simulink model "bloques_motor"  (R2021b)
settings: Solver=FixedStepAuto  StartTime=0.0  StopTime=Tc  FixedStep=Ts  RelTol=1e-3
values from neighbouring files (symbols this model uses):
  a = (Ts/tau) * Kc    (= 0.000110235109441)    [raiz.m]
  a1 = kp + (ki*Tz)    (= 0.0012908137)    [raiz.m]
  b = (Ts/tau) - 1.0    (= -0.999889764891)    [raiz.m]
  b1 = -kp    (= -0.0012852)    [raiz.m]
  Kc = 1.0    (= 1)    [raiz.m]
  sp = -3000    [raiz.m]
  tau = 0.453576    [raiz.m]
  Tz = 0.001    [raiz.m]
settings Model: Creator=yeezvs  LastModifiedBy=yeezvs
settings DataIOCC: ReturnWorkspaceOutputs=off

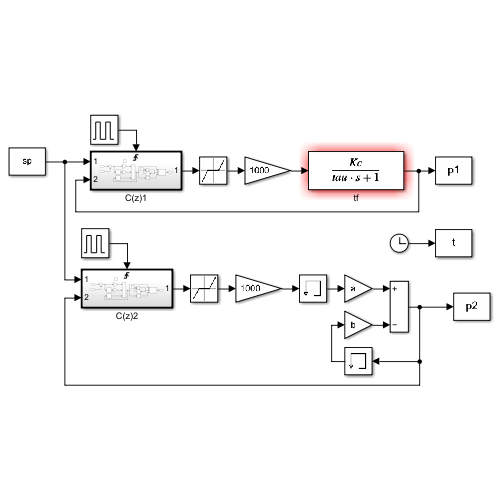
[thumbnail: Simulink's stored preview of the top-level diagram]
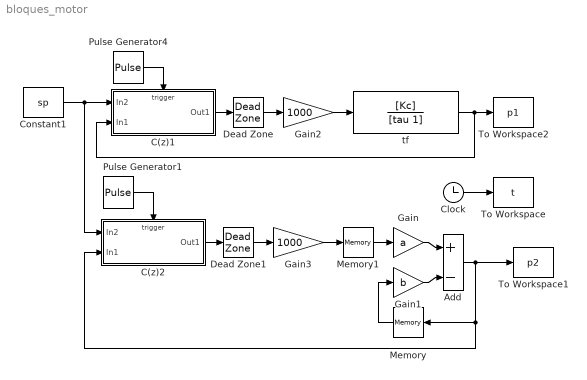
== system bloques_motor ==
  Add : Sum  Inputs=+|-
  C(z)1 : Subsystem  TreatAsAtomicUnit=on
  C(z)2 : Subsystem  TreatAsAtomicUnit=on
  Clock : Clock
  Constant1 : Constant  Value=sp
  Dead Zone : DeadZone  SaturateOnIntegerOverflow=on
  Dead Zone1 : DeadZone  SaturateOnIntegerOverflow=on
  Gain : Gain  Gain=a
  Gain1 : Gain  Gain=b
  Gain2 : Gain  Gain=1000
  Gain3 : Gain  Gain=1000
  Memory : Memory
  Memory1 : Memory
  Pulse Generator1 : DiscretePulseGenerator  PulseType=Time based  Period=Tz  PulseWidth=50
  Pulse Generator4 : DiscretePulseGenerator  PulseType=Time based  Period=Tz  PulseWidth=50
  To Workspace : ToWorkspace  VariableName=t  SampleTime=-1
      settings: Save2DSignal=2-D array (concatenate along first dimension)
  To Workspace1 : ToWorkspace  VariableName=p2  SampleTime=-1
      settings: Save2DSignal=2-D array (concatenate along first dimension)
  To Workspace2 : ToWorkspace  VariableName=p1  SampleTime=-1
      settings: Save2DSignal=2-D array (concatenate along first dimension)
  tf : TransferFcn  Numerator=[Kc]  Denominator=[tau 1]
  wires:
  Clock/1 -> To Workspace/1
  Gain/1 -> Add/1
  Gain1/1 -> Add/2
  Add/1 -> C(z)2/2(In1), Memory/1, To Workspace1/1
  Memory/1 -> Gain1/1
  Memory1/1 -> Gain/1
  tf/1 -> C(z)1/2(In1), To Workspace2/1
  Constant1/1 -> C(z)2/1(In2), C(z)1/1(In2)
  Gain2/1 -> tf/1
  Pulse Generator4/1 -> C(z)1/Trigger
  Pulse Generator1/1 -> C(z)2/Trigger
  Gain3/1 -> Memory1/1
  Dead Zone/1 -> Gain2/1
  C(z)1/1(Out1) -> Dead Zone/1
  C(z)2/1(Out1) -> Dead Zone1/1
  Dead Zone1/1 -> Gain3/1

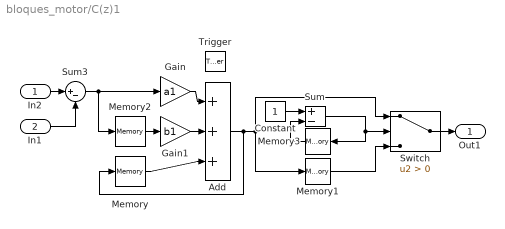
== system bloques_motor/C(z)1 ==
  In2 : Inport
  In1 : Inport  Port=2
  Trigger : TriggerPort  VariantControl=(inherit)
  Add : Sum  Inputs=+|+|+
  Constant : Constant
  Gain : Gain  Gain=a1
  Gain1 : Gain  Gain=b1
  Memory{,1..3} (4 alike) : Memory  InheritSampleTime=on
  Sum : Sum  Inputs=+-  InputSameDT=on  SaturateOnIntegerOverflow=on  OutDataTypeStr=Inherit: Same as first input
  Sum3 : Sum  Inputs=|+-
  Switch : Switch  Criteria=u2 > Threshold
  Out1 : Outport
  wires:
  In2/1 -> Sum3/1
  In1/1 -> Sum3/2
  Gain/1 -> Add/1
  Gain1/1 -> Add/2
  Sum3/1 -> Memory2/1, Gain/1
  Memory2/1 -> Gain1/1
  Memory1/1 -> Switch/3
  Constant/1 -> Sum/1
  Memory3/1 -> Sum/2
  Sum/1 -> Memory3/1, Switch/2
  Add/1 -> Memory/1, Memory1/1, Switch/1
  Switch/1 -> Out1/1
  Memory/1 -> Add/3

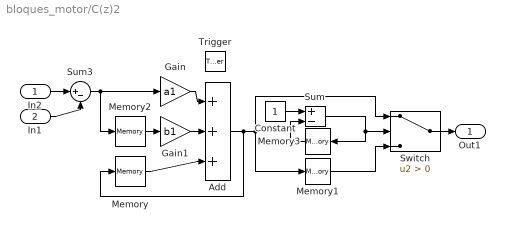
== system bloques_motor/C(z)2 ==
  In2 : Inport
  In1 : Inport  Port=2
  Trigger : TriggerPort  VariantControl=(inherit)
  Add : Sum  Inputs=+|+|+
  Constant : Constant
  Gain : Gain  Gain=a1
  Gain1 : Gain  Gain=b1
  Memory{,1..3} (4 alike) : Memory  InheritSampleTime=on
  Sum : Sum  Inputs=+-  InputSameDT=on  SaturateOnIntegerOverflow=on  OutDataTypeStr=Inherit: Same as first input
  Sum3 : Sum  Inputs=|+-
  Switch : Switch  Criteria=u2 > Threshold
  Out1 : Outport
  wires:
  In2/1 -> Sum3/1
  In1/1 -> Sum3/2
  Gain/1 -> Add/1
  Gain1/1 -> Add/2
  Sum3/1 -> Gain/1, Memory2/1
  Memory2/1 -> Gain1/1
  Memory1/1 -> Switch/3
  Constant/1 -> Sum/1
  Memory3/1 -> Sum/2
  Sum/1 -> Memory3/1, Switch/2
  Add/1 -> Memory/1, Memory1/1, Switch/1
  Switch/1 -> Out1/1
  Memory/1 -> Add/3
